simulink model "v11_memory_block"  (R2019b)
settings: Solver=FixedStepAuto  StartTime=0.0  StopTime=10  FixedStep=1  MaxStep=1  RelTol=1e-3
libraries: SignalEditorBlockLib x1
settings Model: Creator=MARAT  LastModifiedBy=Marat
settings SFSimCC: CustomCodeUndefinedFunction=UseInterfaceOnly

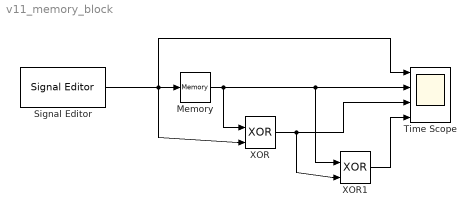
== system v11_memory_block ==
  Memory : Memory
  Signal Editor : SignalEditorBlockLib/Signal Editor  FileName=boolsig.mat  ActiveScenario=Scenario  ActiveSignal=Signal  IsBus=off  OutputBusObjectStr=Bus: BusObject  SampleTime=0  Interpolate=off  ZeroCross=off  OutputAfterFinalValue=Setting to zero  Unit=inherit  PreserveSignalName=on
      settings: SourceProductName=Simulink
  Time Scope : Scope  NumInputPorts=4
  XOR : Logic  Operator=XOR  IconShape=distinctive  AllPortsSameDT=off  OutDataTypeStr=boolean
  XOR1 : Logic  Operator=XOR  IconShape=distinctive  AllPortsSameDT=off  OutDataTypeStr=boolean
  wires:
  Memory/1 -> XOR/1, XOR1/1, Time Scope/2
  Signal Editor/1 -> XOR/2, Time Scope/1, Memory/1
  XOR/1 -> XOR1/2, Time Scope/3
  XOR1/1 -> Time Scope/4
